simulink model "Quaternions_Method_main"  (R2021b)
settings: Solver=ode4  StartTime=0.0  StopTime=Time  FixedStep=1e-2  RelTol=1e-13  AbsTol=1e-8
values from neighbouring files (symbols this model uses):
  a = 8.6251e+06    (= 8625100)    [Main.m]
  c = 299792*10^3    (= 299792000)    [Main.m]
  e = 0.1195    [Main.m]
  f_mag = 5    [Main.m]
  H_0 = sqrt((g_1_0)^2 + (g_1_1)^2 + (h_1_1)^2)    [Main.m]
  i = 0.3815    [Main.m]
  MB = [2000; 0.3; 1; 0.12].*1e-2    [Main.m]
  mr = 1.2 * 0.0001    (= 0.00012)    [Main.m]
  muP = G*Mt    (= 398527110340000)    [Main.m]
  omega_0 = [om_x, om_y, om_z]    [Main.m]
  p_acc = deg2rad(5)    [Main.m]
  RD = 0.1*ones(1,10)    [Main.m]
  RS_MB = 0.5    [Main.m]
  RS_SP = 0.1    [Main.m]
  SP = [2000; 0.3; 1; 0.12].*1e-2    [Main.m]
  theta0 = 0    [Main.m]
  w_E = (2*pi)/(24*3600)    (= 7.27220521664e-05)    [Main.m]
undefined symbols (not defined in the file or in its folder): A_BN_0, A_rw, A_rw_star, k1, k2, magnitude, sig_b, sig_n, T, t_sample
libraries: matrix_library x15, vrlib x8, simulink x2, simulink_extras x1
(part 1 of 5)
settings Model: Creator=dario  LastModifiedBy=hp
settings SolverCC: ZeroCrossAlgorithm=Adaptive  AlgebraicLoopSolver=TrustRegion
settings DataIOCC: Refine=10
settings DebuggingCC: IgnoredZcDiagnostic=none

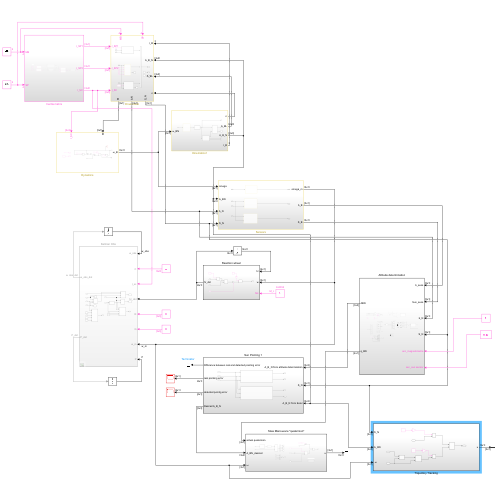
[thumbnail: Simulink's stored preview of the top-level diagram]
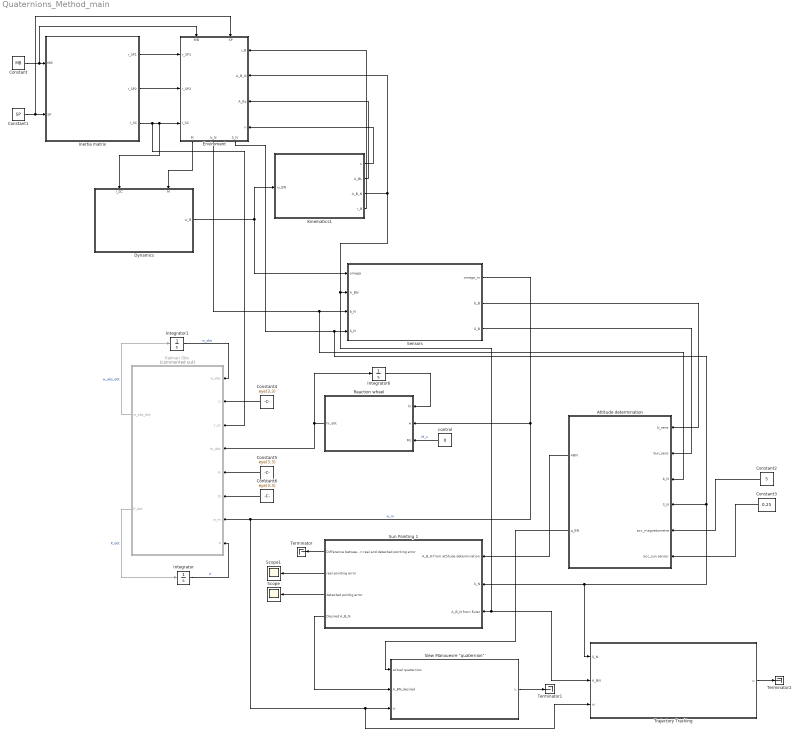
== system Quaternions_Method_main ==
  Attitude determination : Subsystem
  Constant : Constant  Value=MB
  Constant1 : Constant  Value=SP
  Constant2 : Constant  Value=5
  Constant3 : Constant  Value=0.25
  Constant4 : Constant  Value=eye(3,3)
  Constant5 : Constant  Value=eye(3,3)
  Constant6 : Constant  Value=eye(3,3)
  Dynamics : Subsystem
      settings: PortSchema="{\"entries\":[{\"content\":{\"sides\":[{\"content\":{\"connectorIds\":[]},\"type\":\"ConnectorPlacement.EquallySpacedRectSide\",\"uuid\":\"0fb0fd28-732a-45b7-951f-4b0b2306202c\"},{\"content\":{\"connectorIds\":[\"Out1\"],\"side\":\"RIGHT\"},\"type\":\"ConnectorPlacement.EquallySpacedRectSide\",\"uuid\":\"160a6d95-5e8b-4088-9ac4-372e2ef53b1e\"},{\"content\":{\"connectorIds\":[\"In1\",\"In2\"],\"side\":\"TOP\"},\"type\":\"ConnectorPlacement.EquallySpacedRectSide\",\"uuid\":\"bc0d773d-9b3c-40c2-804a-fc9efd6e220c\"}]},\"type\":\"ConnectorPlacement.EquallySpacedConnector\",\"uuid\":\"1f85a25c-c8d4-4d9d-9994-483d99135538\"}],\"packageUris\":[\"http://schema.mathworks.com/mf0/Connector/R2020b\"],\"version\":\"1.0\"}"
  Enviroment : Subsystem
      settings: PortSchema="{\"entries\":[{\"content\":{\"sides\":[{\"content\":{\"connectorIds\":[\"In1\",\"In2\"]},\"type\":\"ConnectorPlacement.EquallySpacedRectSide\",\"uuid\":\"77a65197-c5ef-4c05-af97-bd670bb59a1b\"},{\"content\":{\"connectorIds\":[\"Out1\",\"Out2\",\"Out3\"],\"side\":\"RIGHT\"},\"type\":\"ConnectorPlacement.EquallySpacedRectSide\",\"uuid\":\"f4905732-994b-44e8-915f-1f1165b6d340\"},{\"content\":{\"connectorIds\":[\"In3\",\"In4\",\"In5\"],\"side\":\"TOP\"},\"type\":\"ConnectorPlacement.EquallySpacedRectSide\",\"uuid\":\"dbb628bc-072b-4daa-a580-a056bf799753\"},{\"content\":{\"connectorIds\":[\"In6\",\"In7\",\"In8\",\"In9\"],\"side\":\"BOTTOM\"},\"type\":\"ConnectorPlacement.EquallySpacedRectSide\",\"uuid\":\"e6af6235-b92e-4098-9bbc-91b77f168ead\"}]},\"type\":\"ConnectorPlacement.EquallySpacedConnector\",\"uuid\":\"a4645f0d-8f51-4ba7-9ec5-d423e83ccc17\"}],\"packageUris\":[\"http://schema.mathworks.com/mf0/Connector/R2020b\"],\"version\":\"1.0\"}"
  Inertia matrix : Subsystem
  Integrator : Integrator
  Integrator1 : Integrator
  Integrator6 : Integrator  InitialCondition=[0;0;0;0]
  Kalman Obs : Subsystem  Commented=on
  Kinematics1 : Subsystem
  Reaction wheel : Subsystem
  Scope : Scope
  Scope1 : Scope
  Sensors : Subsystem
  "Slew Manouevre \"quaternion\"" : Subsystem
  Sun Pointing 1 : Subsystem
  Terminator : Terminator
  Terminator1 : Terminator
  Terminator2 : Terminator
  Trajectory Tracking : Subsystem
  control : Constant  Value=0
  wires:
  Constant6/1 -> Kalman Obs/6(Q)
  Sun Pointing 1/1(Difference between real and detected pointing error) -> Terminator/1
  Sun Pointing 1/2(real pointing error) -> Scope1/1
  Sensors/2(b_B) -> Attitude determination/1(b_sens)
  Integrator1/1 -> Kalman Obs/1(w_obs)  "w_obs"
  Enviroment/3(S_N) -> Trajectory Tracking/1(S_N), Sun Pointing 1/2(S_N), Attitude determination/4(S_N), Sensors/4(S_N)
  Inertia matrix/3(I_SC) -> Kalman Obs/3(I_sc), Enviroment/5(I_SC), Dynamics/1(I_SC)
  Integrator6/1 -> Reaction wheel/1(hr)
  Sun Pointing 1/3(detected pointig error) -> Scope/1
  Constant2/1 -> Attitude determination/5(acc_magnetometre)
  Sensors/3(S_B) -> Attitude determination/2(Sun_sens)
  Kalman Obs/1(w_obs_dot) -> Integrator1/1  "w_obs_dot"
  Dynamics/1(ω_B) -> Kinematics1/1(ω_BN), Sensors/1(omega)
  Enviroment/2(b_N) -> Attitude determination/3(b_N), Sensors/3(b_N)
  Constant4/1 -> Kalman Obs/2(C)
  Attitude determination/1(ABN) -> Sun Pointing 1/1(A_B_N from attitude determination)
  Inertia matrix/2(r_SP2) -> Enviroment/4(r_SP2)
  Constant3/1 -> Attitude determination/6(acc_sun sensor)
  Kinematics1/1(n) -> Enviroment/9(n)
  Constant5/1 -> Kalman Obs/5(R)
  control/1 -> Reaction wheel/3(Mc)  "M_c"
  Attitude determination/2(q_BN) -> "Slew Manouevre \"quaternion\""/1(actual quaternion)
  Inertia matrix/1(r_SP1) -> Enviroment/3(r_SP1)
  Constant1/1 -> Inertia matrix/2(SP), Enviroment/2(SP)
  Kinematics1/4(r_B) -> Enviroment/6(r_B)
  Reaction wheel/1(hr_dot) -> Integrator6/1, Kalman Obs/4(hr_dot)
  Sensors/1(omega_m) -> Reaction wheel/2(w), Trajectory Tracking/3(" ω"), "Slew Manouevre \"quaternion\""/3(ω), Kalman Obs/7(w_m)  "w_m"
  Constant/1 -> Inertia matrix/1(MB), Enviroment/1(MB)
  Kinematics1/3(A_B_N) -> Enviroment/7(A_B_N), Trajectory Tracking/2(A_BN), Sun Pointing 1/3(A_B_N from Euler), Sensors/2(A_BN)
  Enviroment/1(M) -> Dynamics/2(M)
  Kalman Obs/2(P_dot) -> Integrator/1  "P_dot"
  Integrator/1 -> Kalman Obs/8(P)  "P"
  Kinematics1/2(A_BL) -> Enviroment/8(A_BL)
  Sun Pointing 1/4(Desired A_B_N) -> "Slew Manouevre \"quaternion\""/2(A_BN_desired)
  "Slew Manouevre \"quaternion\""/1(u) -> Terminator1/1
  Trajectory Tracking/1(u) -> Terminator2/1

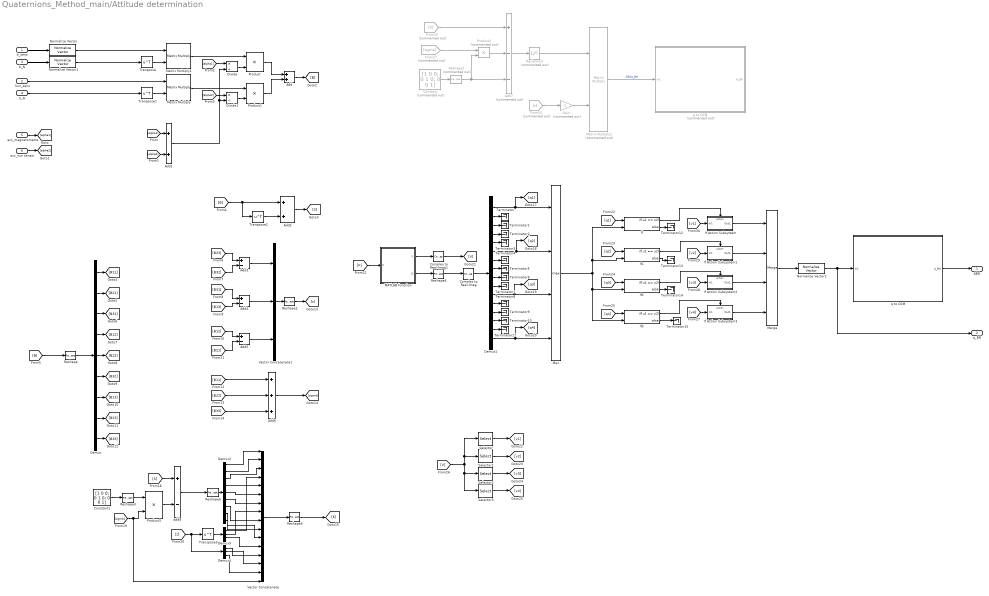
== system Quaternions_Method_main/Attitude determination ==
  b_sens : Inport
  Sun_sens : Inport  Port=2
  b_N : Inport  Port=3
  S_N : Inport  Port=4
  acc_magnetometre : Inport  Port=5
  acc_sun sensor : Inport  Port=6
  Add : Sum
  Add1 : Sum
  Add2 : Sum
  Add{3..5,8} (4 alike) : Sum  Inputs=+-
  Add6 : Sum  Inputs=+++
  Add7 : Sum  Commented=on  Inputs=+--
  Complex to Real-Imag : ComplexToRealImag  Output=Real
  Complex to Real-Imag1 : ComplexToRealImag  Output=Real
  Constant : Constant  Commented=on  Value=[1 0 0; 0 1 0; 0 0 1]  VectorParams1D=off
  Constant1 : Constant  Value=[1 0 0; 0 1 0; 0 0 1]  VectorParams1D=off
  Demux : Demux  Outputs=9
  Demux1 : Demux  Outputs=16
  Demux2 : Demux  Outputs=9
  Demux3 : Demux  Outputs=3
  Demux4 : Demux  Outputs=3
  Divide : Product  Inputs=*/
  Divide1 : Product  Inputs=*/
  From15 : From  Commented=on  GotoTag=z
  From16 : From  Commented=on  GotoTag=S
  From17 : From  Commented=on  GotoTag=sigma
  Gain : Gain  Commented=on  Gain=-1
  If{,1..3} (4 alike) : If  NumInputs=2  IfExpression=u1 == u2
  If Action Subsystem : Subsystem  TreatAsAtomicUnit=on
  If Action Subsystem1 : Subsystem  TreatAsAtomicUnit=on
  If Action Subsystem2 : Subsystem  TreatAsAtomicUnit=on
  If Action Subsystem3 : Subsystem  TreatAsAtomicUnit=on
  MATLAB Function : MATLAB Function  TreatAsAtomicUnit=on
  Matrix Multiply : Product  Multiplication=Matrix(*)
  Matrix Multiply1 : Product  Multiplication=Matrix(*)
  Matrix Multiply2 : Product  Commented=on  Multiplication=Matrix(*)
  Max : MinMax  Function=max  Inputs=4
  Merge : Merge  Inputs=4
  Normalize Vector : vrlib/Utilities/Normalize Vector  maxzero=0
  Normalize Vector1 : vrlib/Utilities/Normalize Vector  maxzero=0
  Normalize Vector2 : vrlib/Utilities/Normalize Vector  maxzero=0
  Product : Product
  Product1 : Product
  Product2 : Product  Commented=on
  Product3 : Product
  Reciprocal : Product  Commented=on  Inputs=/
  Reshape : Reshape
  Reshape1 : Reshape  OutputDimensionality=Column vector (2-D)
  Reshape2 : Reshape  Commented=on  OutputDimensionality=Customize  OutputDimensions=[3,3]
  Reshape3 : Reshape  OutputDimensionality=Customize  OutputDimensions=[3,3]
  Reshape4 : Reshape  OutputDimensionality=Column vector (2-D)
  Reshape5 : Reshape  OutputDimensionality=Column vector (2-D)
  Reshape6 : Reshape  OutputDimensionality=Customize  OutputDimensions=[4,4]
  Selector : Selector  NumberOfDimensions=2  InputPortWidth=3  IndexOptions=Index vector (dialog),Index vector (dialog)  Indices=[1 2 3 4],1  OutputSizes=1,1
  Selector1 : Selector  NumberOfDimensions=2  InputPortWidth=3  IndexOptions=Index vector (dialog),Index vector (dialog)  Indices=[1 2 3 4],2  OutputSizes=1,1
  Selector2 : Selector  NumberOfDimensions=2  InputPortWidth=3  IndexOptions=Index vector (dialog),Index vector (dialog)  Indices=[1 2 3 4],3  OutputSizes=1,1
  Selector3 : Selector  NumberOfDimensions=2  InputPortWidth=3  IndexOptions=Index vector (dialog),Index vector (dialog)  Indices=[1 2 3 4],4  OutputSizes=1,1
  Terminator{,1..15} (16 alike) : Terminator
  Transpose{,1..3} (4 alike) : Math  Operator=transpose  SaturateOnIntegerOverflow=on
  Vector Concatenate : Concatenate  NumInputs=16
  Vector Concatenate1 : Concatenate  NumInputs=3
  g to DCM : Subsystem  Commented=on
  q to DCM : Subsystem
  ABN : Outport
  q_BN : Outport  Port=2
  wires:
  b_N/1 -> Normalize Vector1/1
  S_N/1 -> Transpose1/1
  Sun_sens/1 -> Matrix Multiply/1
  Transpose1/1 -> Matrix Multiply/2
  Transpose/1 -> Matrix Multiply1/2
  b_sens/1 -> Normalize Vector/1
  Matrix Multiply1/1 -> Product/1
  Product/1 -> Add/1
  Divide/1 -> Product/2
  Divide1/1 -> Product1/2
  Product1/1 -> Add/2
  Matrix Multiply/1 -> Product1/1
  Add1/1 -> Divide/2, Divide1/2
  acc_magnetometre/1 -> [alpha1]
  acc_sun sensor/1 -> [alpha2]
  [alpha1] -> Add1/1
  [alpha2] -> Add1/2
  [alpha2] -> Divide1/1
  [alpha1] -> Divide/1
  Add/1 -> [B]
  [B] -> Transpose2/1, Add2/1
  Transpose2/1 -> Add2/2
  Add2/1 -> [S]
  [B] -> Reshape/1
  Reshape/1 -> Demux/1
  Demux/1 -> [B11]
  Demux/2 -> [B21]
  Demux/3 -> [B31]
  Demux/4 -> [B12]
  Demux/5 -> [B22]
  Demux/6 -> [B32]
  Demux/7 -> [B13]
  Demux/8 -> [B23]
  Demux/9 -> [B33]
  [B23] -> Add3/1
  [B32] -> Add3/2
  [B31] -> Add4/1
  [B13] -> Add4/2
  [B12] -> Add5/1
  [B21] -> Add5/2
  Add3/1 -> Vector Concatenate1/1
  Add4/1 -> Vector Concatenate1/2
  Add5/1 -> Vector Concatenate1/3
  Vector Concatenate1/1 -> Reshape1/1
  Reshape1/1 -> [z]
  [B11] -> Add6/1
  [B22] -> Add6/2
  [B33] -> Add6/3
  Add6/1 -> [sigma]
  From15/1 -> Gain/1
  Constant/1 -> Reshape2/1
  From17/1 -> Product2/1
  Reshape2/1 -> Add7/3, Product2/2
  From16/1 -> Add7/1
  Product2/1 -> Add7/2
  Add7/1 -> Reciprocal/1
  Reciprocal/1 -> Matrix Multiply2/1
  Gain/1 -> Matrix Multiply2/2
  Matrix Multiply2/1 -> g to DCM/1(In1)  "Gibbs_BN"
  Constant1/1 -> Reshape3/1
  Reshape3/1 -> Product3/1
  [sigma] -> Vector Concatenate/16, Product3/2
  Product3/1 -> Add8/2
  [S] -> Add8/1
  Add8/1 -> Reshape5/1
  MATLAB Function/2(D) -> Reshape4/1
  Demux1/2 -> Terminator/1
  Demux1/3 -> Terminator1/1
  Demux1/4 -> Terminator2/1
  Demux1/5 -> Terminator3/1
  Demux1/6 -> [q2], Max/2
  Demux1/7 -> Terminator4/1
  Demux1/8 -> Terminator5/1
  Demux1/9 -> Terminator6/1
  Demux1/10 -> Terminator7/1
  Demux1/11 -> [q3], Max/3
  Demux1/16 -> [q4], Max/4
  Demux1/12 -> Terminator8/1
  Demux1/13 -> Terminator9/1
  Demux1/14 -> Terminator10/1
  Demux1/15 -> Terminator11/1
  Reshape4/1 -> Complex to Real-Imag/1
  Max/1 -> If3/2, If2/2, If1/2, If/2
  Demux1/1 -> [q1], Max/1
  [q1] -> If/1
  [q2] -> If1/1
  [q4] -> If3/1
  [q3] -> If2/1
  MATLAB Function/1(V) -> Complex to Real-Imag1/1
  Selector1/1 -> [v2]
  Selector3/1 -> [v4]
  Selector2/1 -> [v3]
  Selector/1 -> [v1]
  [V] -> Selector/1, Selector1/1, Selector3/1, Selector2/1
  If/1 -> If Action Subsystem/Action
  If/2 -> Terminator12/1
  If1/2 -> Terminator13/1
  If2/2 -> Terminator14/1
  If3/2 -> Terminator15/1
  If Action Subsystem/1(Out1) -> Merge/1
  If1/1 -> If Action Subsystem1/Action
  If2/1 -> If Action Subsystem2/Action
  If3/1 -> If Action Subsystem3/Action
  If Action Subsystem3/1(Out1) -> Merge/4
  If Action Subsystem2/1(Out1) -> Merge/3
  If Action Subsystem1/1(Out1) -> Merge/2
  [v4] -> If Action Subsystem3/1(In1)
  [v1] -> If Action Subsystem/1(In1)
  [v2] -> If Action Subsystem1/1(In1)
  Normalize Vector/1 -> Matrix Multiply1/1
  Normalize Vector1/1 -> Transpose/1
  [v3] -> If Action Subsystem2/1(In1)
  q to DCM/1(A_BN) -> ABN/1
  Merge/1 -> Normalize Vector2/1
  Reshape5/1 -> Demux2/1
  Demux2/1 -> Vector Concatenate/1
  Demux2/2 -> Vector Concatenate/2
  Demux2/3 -> Vector Concatenate/3
  [z] -> Demux4/1, Transpose3/1
  Transpose3/1 -> Demux3/1
  Demux3/1 -> Vector Concatenate/4
  Demux2/4 -> Vector Concatenate/5
  Demux2/5 -> Vector Concatenate/6
  Demux2/6 -> Vector Concatenate/7
  Demux3/2 -> Vector Concatenate/8
  Demux2/7 -> Vector Concatenate/9
  Demux2/8 -> Vector Concatenate/10
  Demux2/9 -> Vector Concatenate/11
  Demux3/3 -> Vector Concatenate/12
  Demux4/2 -> Vector Concatenate/14
  Demux4/1 -> Vector Concatenate/13
  Demux4/3 -> Vector Concatenate/15
  Vector Concatenate/1 -> Reshape6/1
  Reshape6/1 -> [K]
  Complex to Real-Imag/1 -> Demux1/1
  Normalize Vector2/1 -> q_BN/1, q to DCM/1(In1)
  Complex to Real-Imag1/1 -> [V]
  [K] -> MATLAB Function/1(K)

== system Quaternions_Method_main/Dynamics ==
  I_SC : Inport
  M : Inport  Port=2
  Constant7 : Constant  Value=omega_0
  Cross Product : vrlib/Utilities/Cross Product
  Gain5 : Gain  Gain=-1
  Integrator4 : Integrator  InitialConditionSource=external  InitialCondition=omega_0
  Product6 : Product  Multiplication=Matrix(*)
  Product7 : Product  Multiplication=Matrix(*)
  Reciprocal : Product  Inputs=/  Multiplication=Matrix(*)
  Scope : Scope
  Sum2 : Sum
  Terminator : Terminator
  ω_B : Outport
  wires:
  Sum2/1 -> Product7/2
  Product6/1 -> Cross Product/2
  Product7/1 -> Terminator/1, Integrator4/1
  Cross Product/1 -> Gain5/1
  Gain5/1 -> Sum2/1
  Integrator4/1 -> Scope/1, Cross Product/1, Product6/2, ω_B/1
  I_SC/1 -> [I_SC]
  [I_SC] -> Product6/1
  [I_SC] -> Reciprocal/1
  Reciprocal/1 -> Product7/1
  Constant7/1 -> [w_0]
  [w_0] -> Integrator4/2
  M/1 -> Sum2/2

== system Quaternions_Method_main/Enviroment ==
  MB : Inport
  SP : Inport  Port=2
  r_SP1 : Inport  Port=3
  r_SP2 : Inport  Port=4
  I_SC : Inport  Port=5
  r_B : Inport  Port=6
  A_B_N : Inport  Port=7
  A_BL : Inport  Port=8
  n : Inport  Port=9
  Constant : Constant  Value=6371.2*1e3
  Gravity gradient torque : Subsystem
  "Magnetic torque " : Subsystem
  Solar Radiation Perturbation : Subsystem
  Sum : Sum  Inputs=+|+|+
  M : Outport
  b_N : Outport  Port=2
  S_N : Outport  Port=3
  wires:
  A_B_N/1 -> "Magnetic torque "/3(A_B_N), Solar Radiation Perturbation/1(A_B_N)
  MB/1 -> Solar Radiation Perturbation/2(MB)
  SP/1 -> Solar Radiation Perturbation/3(SP)
  r_SP1/1 -> Solar Radiation Perturbation/4(r_SP1)
  r_SP2/1 -> Solar Radiation Perturbation/5(r_SP2)
  Sum/1 -> M/1
  Solar Radiation Perturbation/1(M_SRP) -> Sum/2
  "Magnetic torque "/1(M) -> Sum/3
  r_B/1 -> "Magnetic torque "/1(r_B)
  Constant/1 -> "Magnetic torque "/2(R)
  Gravity gradient torque/1(M_GG) -> Sum/1
  I_SC/1 -> Gravity gradient torque/1(I)
  n/1 -> Gravity gradient torque/3(n)
  A_BL/1 -> Gravity gradient torque/2(A_BL)
  "Magnetic torque "/2(b_N) -> [b_N]
  [b_N] -> b_N/1
  Solar Radiation Perturbation/2(S_N) -> [S_N]
  [S_N] -> S_N/1

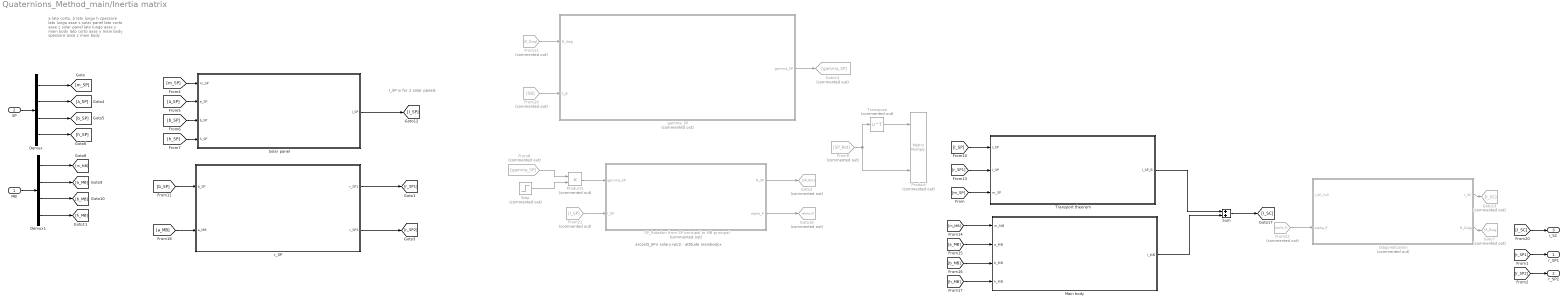
== system Quaternions_Method_main/Inertia matrix ==
  note: I_SP is for 2 solar panels
  note: arcos(S_B*n solary)-pi/2 - attitude mainbodyx
  note: a lato corto, b lato lungo h spessore
      | lato lungo asse x solar panel
      | lato corto asse z solar panel
      | lato lungo asse y main body
      | lato corto asse x main body
      | spessore asse z main body
  MB : Inport
  SP : Inport  Port=2
  Demux : Demux
  Demux1 : Demux
  Diagonalization : Subsystem  Commented=on
  From12 : From  Commented=on  GotoTag=R_Diag
  From19 : From  Commented=on  GotoTag=SB
  From21 : From  Commented=on  GotoTag=I_SP
  From22 : From  Commented=on  GotoTag=alpha_P
  From8 : From  Commented=on  GotoTag=gamma_SP
  From9 : From  Commented=on  GotoTag=SP_Rot
  Goto13 : Goto  Commented=on  GotoTag=I_SC
  Goto14 : Goto  Commented=on  GotoTag=gamma_SP
  Goto16 : Goto  Commented=on  GotoTag=alpha_P
  Goto2 : Goto  Commented=on  GotoTag=SP_Rot
  Goto7 : Goto  Commented=on  GotoTag=R_Diag
  Main body : Subsystem
  Product : Product  Commented=on  Inputs=3  Multiplication=Matrix(*)
  Product1 : Product  Commented=on
  SP_Rotation from SP principal to MB principal : Subsystem  Commented=on
  Solar panel : Subsystem
  Step : Step  Commented=on  Time=1e-3  SampleTime=0
  Sum : Sum
  Transport theorem : Subsystem
  Transpose : Math  Commented=on  Operator=transpose  SaturateOnIntegerOverflow=on
  gamma_SP : Subsystem  Commented=on
  r_SP : Subsystem
  r_SP1 : Outport
  r_SP2 : Outport  Port=2
  I_SC : Outport  Port=3
  wires:
  MB/1 -> Demux1/1
  Demux/1 -> [m_SP]
  SP_Rotation from SP principal to MB principal/1(R_SP) -> Goto2/1
  Transpose/1 -> Product/1
  Transport theorem/1(I_SP_B) -> Sum/1
  [r_SP1] -> Transport theorem/2(r_SP)
  Main body/1(I_MB) -> Sum/2
  [m_SP] -> Transport theorem/3(m_SP)
  r_SP/1(r_SP1) -> [r_SP1]
  [r_SP1] -> r_SP1/1
  [r_SP2] -> r_SP2/1
  r_SP/2(r_SP2) -> [r_SP2]
  Demux/2 -> [a_SP]
  Demux/3 -> [b_SP]
  Demux/4 -> [h_SP]
  [a_SP] -> Solar panel/2(a_SP)
  [b_SP] -> Solar panel/3(b_SP)
  [m_SP] -> Solar panel/1(m_SP)
  [h_SP] -> Solar panel/4(h_SP)
  From9/1 -> Transpose/1, Product/3
  [b_SP] -> r_SP/1(b_SP)
  Demux1/4 -> [h_MB]
  Demux1/3 -> [b_MB]
  Demux1/2 -> [a_MB]
  Demux1/1 -> [m_MB]
  [m_MB] -> Main body/1(m_MB)
  [a_MB] -> Main body/2(a_MB)
  [b_MB] -> Main body/3(b_MB)
  [h_MB] -> Main body/4(h_MB)
  [a_MB] -> r_SP/2(a_MB)
  Solar panel/1(I_SP) -> [I_SP]
  Product1/1 -> SP_Rotation from SP principal to MB principal/1(gamma_SP)
  From8/1 -> Product1/1
  Step/1 -> Product1/2
  SP/1 -> Demux/1
  Diagonalization/2(R_Diag) -> Goto7/1
  From12/1 -> gamma_SP/1(R_diag)
  From19/1 -> gamma_SP/2(S_B)
  Diagonalization/1(I_SC) -> Goto13/1
  [I_SC] -> I_SC/1
  gamma_SP/1(gamma_SP) -> Goto14/1
  From21/1 -> SP_Rotation from SP principal to MB principal/2(I_SP)
  SP_Rotation from SP principal to MB principal/2(alpha_P) -> Goto16/1
  From22/1 -> Diagonalization/2(alpha_P)
  [I_SP] -> Transport theorem/1(I_SP)
  Sum/1 -> [I_SC]

== system Quaternions_Method_main/Kalman Obs ==
  w_obs : Inport
  C : Inport  Port=2
  I_sc : Inport  Port=3
  hr_dot : Inport  Port=4
  R : Inport  Port=5
  Q : Inport  Port=6
  w_m : Inport  Port=7
  P : Inport  Port=8
  Subsystem : Subsystem
  Subsystem1 : Subsystem
  Subsystem2 : Subsystem
  Subsystem3 : Subsystem
  Subsystem4 : Subsystem
  Subsystem5 : Subsystem
  w_obs_dot : Outport
  P_dot : Outport  Port=2
  wires:
  I_sc/1 -> Subsystem4/3(I_sc), Subsystem/1(I_SC)
  Subsystem/1(K) -> Subsystem4/1(K), Subsystem1/2(K)  "K"
  w_obs/1 -> Subsystem4/2(w_obs), Subsystem1/1(w_obs), Subsystem3/4(w_obs)
  Subsystem1/1(A) -> [A]
  C/1 -> Subsystem3/3(C), [C], Subsystem2/1(C)
  P/1 -> Subsystem5/1(P), Subsystem2/2(P)
  R/1 -> Subsystem2/3(R), [R]
  Subsystem2/1(L) -> Subsystem3/1(L)  "L"
  w_m/1 -> Subsystem3/2(w_m)
  Subsystem3/1(Ly) -> [Ly]
  Subsystem4/1(w_obs_dot) -> w_obs_dot/1
  hr_dot/1 -> Subsystem4/4(hr_dot)
  [Ly] -> Subsystem4/5(Ly)
  [A] -> Subsystem5/2(A)
  Q/1 -> Subsystem5/3(Q)
  [C] -> Subsystem5/4(C)
  [R] -> Subsystem5/5(R)
  Subsystem5/1(P_dot) -> P_dot/1

== system Quaternions_Method_main/Kinematics1 ==
  ω_BN : Inport
  Creazione Matrice A_BN : Subsystem
  Creazione quaternione : Subsystem
  Orbit Propagation : Subsystem
  Relative_Attitude : Subsystem
  n : Outport
  A_BL : Outport  Port=2
  A_B_N : Outport  Port=3
  r_B : Outport  Port=4
  wires:
  Creazione Matrice A_BN/1(A_BN) -> A_B_N/1, Relative_Attitude/1(A_BN), Orbit Propagation/1(A_BN)
  ω_BN/1 -> Creazione quaternione/1(ω_BN)
  Creazione quaternione/1(q_normalizzato) -> Creazione Matrice A_BN/1(q_normalizzato)
  Relative_Attitude/1(A_BL) -> A_BL/1
  Orbit Propagation/2(n) -> n/1
  Orbit Propagation/3(rB) -> r_B/1
  Orbit Propagation/1(theta) -> Relative_Attitude/2(theta)
  Relative_Attitude/2(A_L/N) -> [A_LN]

== system Quaternions_Method_main/Reaction wheel ==
  hr : Inport
  w : Inport  Port=2
  Mc : Inport  Port=3
  A : Constant  Value=A_rw
  A_star : Constant  Value=A_rw_star
  Cross Product : matrix_library/Cross Product
      settings: SourceProductBaseCode=SL
  Gain : Gain  Gain=-1
  Matrix Multiply : Product  Multiplication=Matrix(*)
  Matrix Multiply1 : Product  Multiplication=Matrix(*)
  Sum : Sum  Inputs=|++
  hr_dot : Outport
  wires:
  hr/1 -> Matrix Multiply/2
  A/1 -> Matrix Multiply/1
  w/1 -> Cross Product/1
  Matrix Multiply/1 -> Cross Product/2
  Cross Product/1 -> Sum/1
  Mc/1 -> Sum/2
  Sum/1 -> Matrix Multiply1/2
  A_star/1 -> Gain/1
  Gain/1 -> Matrix Multiply1/1
  Matrix Multiply1/1 -> hr_dot/1

== system Quaternions_Method_main/Sensors ==
  omega : Inport
  A_BN : Inport  Port=2
  b_N : Inport  Port=3
  S_N : Inport  Port=4
  Gyroscopes : Subsystem
  Magnetometer1 : Subsystem
  Sun sensor : Subsystem
  omega_m : Outport
  b_B : Outport  Port=2
  S_B : Outport  Port=3
  wires:
  omega/1 -> Gyroscopes/1(omega)
  Gyroscopes/1(omega_m) -> omega_m/1
  b_N/1 -> Magnetometer1/2(b_N)
  Magnetometer1/1(b_B) -> b_B/1
  Sun sensor/1(S_B) -> S_B/1
  A_BN/1 -> Sun sensor/2(A_BN), Magnetometer1/1(A_BN)
  S_N/1 -> Sun sensor/1(S_N)

== system Quaternions_Method_main/Slew Manouevre "quaternion" ==
  note: here I compute the derivative wrt q4e
      | of the function H(q4e) = 1 - q4e^2
  actual quaternion : Inport
  A_BN_desired : Inport  Port=2
  ω : Inport  Port=3
  A_BN to quaternion : Subsystem
  Constant : Constant  Value=k1
  Constant1 : Constant  Value=k2
  Creation of Q_euler1 : Subsystem
  Demux : Demux
  Gain : Gain  Gain=-1
  Gain1 : Gain  Gain=-2
  Mux : Mux  Inputs=3
  Product : Product  Multiplication=Matrix(*)
  Product1 : Product
  Product2 : Product  Inputs=3
  Reshape : Reshape  OutputDimensionality=Column vector (2-D)
  Sum : Sum  Inputs=|+|+|
  d/dq4e(H(q4e)) : Subsystem  Commented=on
  u : Outport
  wires:
  actual quaternion/1 -> Product/2
  Creation of Q_euler1/1(Q_desired) -> Product/1
  A_BN_desired/1 -> A_BN to quaternion/1(" A_BN_Desiderd")
  A_BN to quaternion/1(q_desiderd) -> Creation of Q_euler1/1(q_desired)
  Constant/1 -> Gain/1
  Gain/1 -> Product1/1
  ω/1 -> Product1/2
  Constant1/1 -> Product2/1
  [q_error] -> Product2/3
  Product1/1 -> Sum/1
  Product2/1 -> Sum/2
  Sum/1 -> u/1
  Product/1 -> Demux/1
  Demux/1 -> [qe1]
  Demux/4 -> [qe4]
  Demux/3 -> [qe3]
  Demux/2 -> [qe2]
  [qe1] -> Mux/1
  [qe2] -> Mux/2
  [qe3] -> Mux/3
  Mux/1 -> Reshape/1
  Reshape/1 -> [q_error]
  [qe4] -> Gain1/1
  Gain1/1 -> Product2/2

== system Quaternions_Method_main/Sun Pointing 1 ==
  A_B_N from attitude determination : Inport
  S_N : Inport  Port=2
  A_B_N from Euler : Inport  Port=3
  Pointing error with DCM : Subsystem
  Pointing error with quaternions : Subsystem
  Difference between real and detected pointing error : Outport
  real pointing error : Outport  Port=2
  detected pointig error : Outport  Port=3
  Desired A_B_N : Outport  Port=4
  wires:
  A_B_N from attitude determination/1 -> Pointing error with quaternions/1(A_B_N from attitude determination), Pointing error with DCM/3(A_B_N from Euler)
  S_N/1 -> Pointing error with quaternions/2(S_N), Pointing error with DCM/2(S_N)
  A_B_N from Euler/1 -> Pointing error with quaternions/3(A_B_N from Euler), Pointing error with DCM/1(A_B_N from attitude determination)
  Pointing error with DCM/1(Difference between real and detected pointing error) -> Difference between real and detected pointing error/1
  Pointing error with quaternions/2(detected pointing error) -> detected pointig error/1
  Pointing error with quaternions/1(real pointing error) -> real pointing error/1
  Pointing error with DCM/2(Desired A_B_N) -> Desired A_B_N/1

== system Quaternions_Method_main/Trajectory Tracking ==
  S_N : Inport
  A_BN : Inport  Port=2
  " ω" : Inport  Port=3
  Constant : Constant  Value=k1
  Constant1 : Constant  Value=k2
  Cross Product : matrix_library/Cross Product
      settings: SourceProductBaseCode=SL
  Gain : Gain  Gain=-1
  Gain1 : Gain  Gain=-1
  Matrix Multiply : Product  Multiplication=Matrix(*)
  Product : Product
  Product1 : Product
  Sum : Sum  Inputs=|+|+|
  u : Outport
  wires:
  S_N/1 -> Cross Product/2, Matrix Multiply/2
  A_BN/1 -> Matrix Multiply/1
  Constant/1 -> Gain/1
  Constant1/1 -> Gain1/1
  Matrix Multiply/1 -> Cross Product/1
  Cross Product/1 -> Product/2
  Gain1/1 -> Product/1
  Gain/1 -> Product1/1
  " ω"/1 -> Product1/2
  Product1/1 -> Sum/1
  Product/1 -> Sum/2
  Sum/1 -> u/1

== system Quaternions_Method_main/Attitude determination/If Action Subsystem ==
  In1 : Inport
  Action Port : ActionPort  ActionPortLabel=if(u1 == u2)
  Out1 : Outport
  wires:
  In1/1 -> Out1/1

== system Quaternions_Method_main/Attitude determination/If Action Subsystem1 ==
  In1 : Inport
  Action Port : ActionPort  ActionPortLabel=if(u1 == u2)
  Out1 : Outport
  wires:
  In1/1 -> Out1/1

== system Quaternions_Method_main/Attitude determination/If Action Subsystem2 ==
  In1 : Inport
  Action Port : ActionPort  ActionPortLabel=if(u1 == u2)
  Out1 : Outport
  wires:
  In1/1 -> Out1/1

== system Quaternions_Method_main/Attitude determination/If Action Subsystem3 ==
  In1 : Inport
  Action Port : ActionPort  ActionPortLabel=if(u1 == u2)
  Out1 : Outport
  wires:
  In1/1 -> Out1/1

== system Quaternions_Method_main/Attitude determination/g to DCM ==
  In1 : Inport
  A_BN : Outport
  wires:
  In1/1 -> A_BN/1

== system Quaternions_Method_main/Attitude determination/q to DCM ==
  In1 : Inport
  Add : Sum  Inputs=+-
  Add1 : Sum  Inputs=++-
  Constant : Constant  Value=[1 0 0; 0 1 0; 0 0 1]  VectorParams1D=off
  Demux : Demux
  Gain : Gain  Gain=2
  Gain1 : Gain  Gain=2
  Matrix Multiply : Product  Multiplication=Matrix(*)
  Matrix Multiply2 : Product  Multiplication=Matrix(*)
  Mux : Mux  Inputs=3
  Product : Product
  Product1 : Product
  Reshape : Reshape  OutputDimensionality=Column vector (2-D)
  Reshape1 : Reshape  OutputDimensionality=Customize  OutputDimensions=[3,3]
  Square : Math  Operator=square  SaturateOnIntegerOverflow=on
  Transpose : Math  Operator=transpose  SaturateOnIntegerOverflow=on
  Transpose1 : Math  Operator=transpose  SaturateOnIntegerOverflow=on
  q_cross : Subsystem
  A_BN : Outport
  wires:
  In1/1 -> Demux/1
  Demux/4 -> [q4]
  Demux/1 -> [q1]
  Demux/2 -> [q2]
  Demux/3 -> [q3]
  [q4] -> Square/1
  [q2] -> Mux/2
  [q3] -> Mux/3
  [q1] -> Mux/1
  Mux/1 -> Reshape/1
  Reshape/1 -> [q_vect]
  [q_vect] -> Matrix Multiply/2, Transpose/1
  Transpose/1 -> Matrix Multiply/1
  Matrix Multiply/1 -> Add/2
  Square/1 -> Add/1
  Constant/1 -> Reshape1/1
  Reshape1/1 -> Product1/2
  Product1/1 -> Add1/1
  Matrix Multiply2/1 -> Gain/1
  Gain/1 -> Add1/2
  Transpose1/1 -> Matrix Multiply2/2
  [q_vect] -> Transpose1/1, Matrix Multiply2/1
  Gain1/1 -> Add1/3
  Product/1 -> Gain1/1
  [q4] -> Product/2
  q_cross/1(q_cross) -> Product/1
  Add1/1 -> A_BN/1
  [q_vect] -> q_cross/1(q_vect)
  Add/1 -> Product1/1

== system Quaternions_Method_main/Enviroment/Gravity gradient torque ==
  I : Inport
  A_BL : Inport  Port=2
  n : Inport  Port=3
  Constant1 : Constant  Value=[1 0 0]
  Demux : Demux  Outputs=9
  Demux1 : Demux  Outputs=3
  Matrix Multiply : Product  Multiplication=Matrix(*)
  Mux : Mux  Inputs=3
  Product{1..9} (9 alike) : Product
  Reshape : Reshape  OutputDimensionality=Column vector (2-D)
  Reshape1 : Reshape  OutputDimensionality=Column vector (2-D)
  Sum : Sum  Inputs=+-
  Sum1 : Sum  Inputs=+-
  Sum2 : Sum  Inputs=+-
  Terminator{,1..5} (6 alike) : Terminator
  M_GG : Outport
  wires:
  Demux/4 -> Terminator2/1
  n/1 -> Product3/2, Product1/2, Product2/2
  Demux1/1 -> Product5/2, Product7/2
  Demux/2 -> Terminator/1
  Product6/1 -> Product9/1
  Sum/1 -> Product1/1
  Product1/1 -> Product6/1
  Demux/7 -> Terminator4/1
  Demux1/3 -> Product6/2, Product8/2
  Demux/1 -> Sum1/1
  Product5/1 -> Product8/1
  Demux/3 -> Terminator1/1
  I/1 -> Reshape1/1
  Matrix Multiply/1 -> Demux1/1
  Demux/9 -> Sum2/2, Sum1/2, Sum/1
  Constant1/1 -> Reshape/1
  Sum1/1 -> Product2/1
  Sum2/1 -> Product3/1
  Product7/1 -> Mux/3
  Mux/1 -> M_GG/1
  Demux/5 -> Sum/2, Sum2/1
  Demux/8 -> Terminator5/1
  A_BL/1 -> Matrix Multiply/1
  Product4/1 -> Product7/1
  Product8/1 -> Mux/2
  Demux/6 -> Terminator3/1
  Demux1/2 -> Product4/2, Product9/2
  Product2/1 -> Product5/1
  Product9/1 -> Mux/1
  Product3/1 -> Product4/1
  Reshape/1 -> Matrix Multiply/2
  Reshape1/1 -> Demux/1

== system Quaternions_Method_main/Enviroment/Magnetic torque  ==
  r_B : Inport
  R : Inport  Port=2
  A_B_N : Inport  Port=3
  Creation of parasitic torque : Subsystem
  Cross Product : matrix_library/Cross Product
      settings: SourceProductBaseCode=SL
  Magnetic torque in body frame : Subsystem
  Matrix Multiply : Product  Multiplication=Matrix(*)
  M : Outport
  b_N : Outport  Port=2
  wires:
  R/1 -> Magnetic torque in body frame/3(R)
  A_B_N/1 -> Magnetic torque in body frame/1(A_B_N), Matrix Multiply/1
  Magnetic torque in body frame/1(b_B) -> Cross Product/2
  Cross Product/1 -> M/1
  Matrix Multiply/1 -> Magnetic torque in body frame/2(r_N)
  r_B/1 -> Matrix Multiply/2
  Creation of parasitic torque/1(m) -> Cross Product/1
  Magnetic torque in body frame/2(b_N) -> b_N/1

== system Quaternions_Method_main/Enviroment/Solar Radiation Perturbation ==
  A_B_N : Inport
  MB : Inport  Port=2
  SP : Inport  Port=3
  r_SP1 : Inport  Port=4
  r_SP2 : Inport  Port=5
  Force1 : Subsystem
  Normalize Vector : vrlib/Utilities/Normalize Vector  maxzero=0
  Sum forces : Subsystem
      settings: PortSchema="{\"entries\":[{\"content\":{\"sides\":[{\"content\":{\"connectorIds\":[\"In1\",\"In2\",\"In3\",\"In4\",\"In5\",\"In6\",\"In7\"]},\"type\":\"ConnectorPlacement.EquallySpacedRectSide\",\"uuid\":\"5acb7d4f-0337-4224-9758-4598a3a00165\"},{\"content\":{\"connectorIds\":[\"Out1\"],\"side\":\"RIGHT\"},\"type\":\"ConnectorPlacement.EquallySpacedRectSide\",\"uuid\":\"e6f98c05-9b5f-4378-b9e9-dabff353d596\"},{\"content\":{\"connectorIds\":[],\"side\":\"TOP\"},\"type\":\"ConnectorPlacement.EquallySpacedRectSide\",\"uuid\":\"88e90ea7-7ab4-48d4-8e3b-8712b3a0b993\"},{\"content\":{\"connectorIds\":[\"In8\"],\"side\":\"BOTTOM\"},\"type\":\"ConnectorPlacement.EquallySpacedRectSide\",\"uuid\":\"ececea6a-2c27-462e-a638-503b4beb3cbf\"}]},\"type\":\"ConnectorPlacement.EquallySpacedConnector\",\"uuid\":\"86da1db6-5ce7-4d9e-9b5c-c43957a7360d\"}],\"packageUris\":[\"http://schema.mathworks.com/mf0/Connector/R2020b\"],\"version\":\"1.0\"}"
  Sun position body : Subsystem
  M_SRP : Outport
  S_N : Outport  Port=2
  wires:
  A_B_N/1 -> Sun position body/1(A_B_N)
  Sun position body/1(S_B) -> Normalize Vector/1
  Normalize Vector/1 -> Force1/1(SB)
  Force1/3(A_MB) -> Sum forces/5(A_MB)
  Force1/1(F_MB) -> Sum forces/3(F_MB)
  r_SP1/1 -> Sum forces/1(r_SP1)
  r_SP2/1 -> Sum forces/2(r_SP2)
  Force1/5(prodscal_SP1) -> Sum forces/7(prodscal_SP (tra norm e sun direction))
  Force1/4(prodsca_MB) -> Sum forces/6(prodscal_MB(tra norm e sun direction))
  Sum forces/1(M_SRP) -> M_SRP/1
  MB/1 -> [MB]
  SP/1 -> [SP]
  [MB] -> Force1/2(MB)
  [SP] -> Force1/3(SP)
  [MB] -> Sum forces/8(MB)
  Force1/2(F_SP) -> Sum forces/4(F_SP)
  Sun position body/2(S_N) -> [S_N]
  [S_N] -> S_N/1

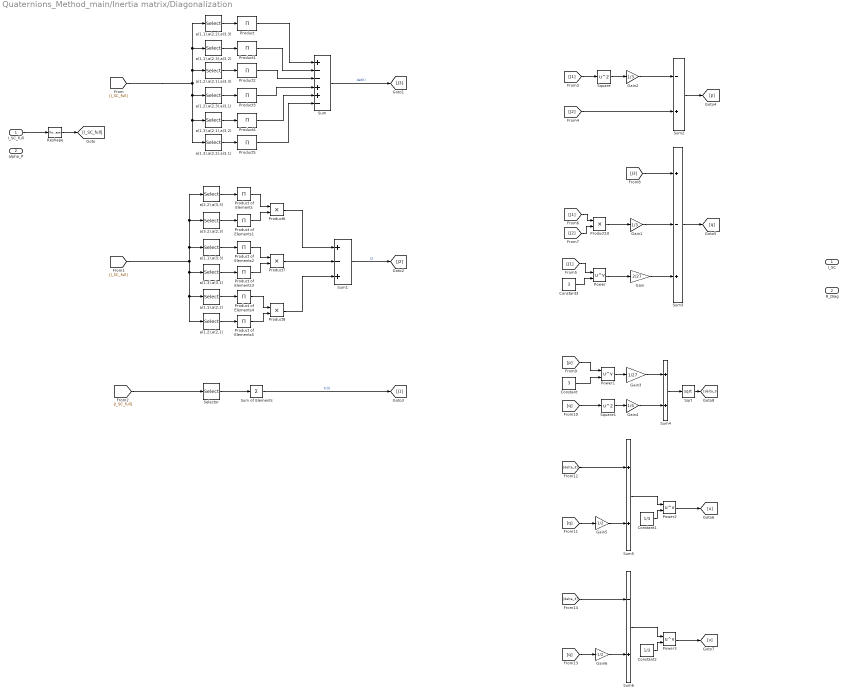
== system Quaternions_Method_main/Inertia matrix/Diagonalization ==
  I_SC_full : Inport
  alpha_P : Inport  Port=2
  Constant : Constant  Value=3
  Constant1 : Constant  Value=1/3
  Constant2 : Constant  Value=1/3
  Constant3 : Constant  Value=3
  Gain : Gain  Gain=2/27
  Gain1 : Gain  Gain=1/3
  Gain2 : Gain  Gain=1/3
  Gain3 : Gain  Gain=1/27
  Gain4 : Gain  Gain=1/4
  Gain5 : Gain  Gain=-1/2
  Gain6 : Gain  Gain=-1/2
  Power{,1..3} (4 alike) : Math  Operator=pow  SaturateOnIntegerOverflow=on
  Product{,1..5} (6 alike) : Product  Inputs=1  SaturateOnIntegerOverflow=on  OutDataTypeStr=Inherit: Same as first input
  Product of Elements{,1..5} (6 alike) : Product  Inputs=*
  Product{6..8,10} (4 alike) : Product
  Reshape : Reshape  OutputDimensionality=Column vector (2-D)
  Selector : Selector  InputPortWidth=9  IndexOptions=Index vector (dialog)  Indices=[1 5 9]  OutputSizes=1
  Sqrt : Sqrt  SaturateOnIntegerOverflow=on
  Square : Math  Operator=square  SaturateOnIntegerOverflow=on
  Square1 : Math  Operator=square  SaturateOnIntegerOverflow=on
  Sum : Sum  Inputs=+--++-  SaturateOnIntegerOverflow=on
  Sum of Elements : Sum  Inputs=+
  Sum1 : Sum  Inputs=+-+
  Sum2 : Sum  Inputs=-+
  Sum3 : Sum  Inputs=+-+
  Sum4 : Sum
  Sum5 : Sum
  Sum6 : Sum  Inputs=-+
  a(1,1),a(2,2) : Selector  InputPortWidth=9  IndexOptions=Index vector (dialog)  Indices=[1 3]  OutputSizes=1
  a(1,1),a(2,2),a(3,3) : Selector  InputPortWidth=9  IndexOptions=Index vector (dialog)  Indices=[1 5 9]  OutputSizes=1
  a(1,1),a(2,3),a(3,2) : Selector  InputPortWidth=9  IndexOptions=Index vector (dialog)  Indices=[1 6 8]  OutputSizes=1
  a(1,2),a(2,1) : Selector  InputPortWidth=9  IndexOptions=Index vector (dialog)  Indices=[1 3]  OutputSizes=1
  a(1,2),a(2,1),a(3,3) : Selector  InputPortWidth=9  IndexOptions=Index vector (dialog)  Indices=[2 4 9]  OutputSizes=1
  a(1,2),a(2,3),a(3,1) : Selector  InputPortWidth=9  IndexOptions=Index vector (dialog)  Indices=[3 4 8]  OutputSizes=1
  a(1,3),a(2,1),a(3,2) : Selector  InputPortWidth=9  IndexOptions=Index vector (dialog)  Indices=[2 6 7]  OutputSizes=1
  a(1,3),a(2,2),a(3,1) : Selector  InputPortWidth=9  IndexOptions=Index vector (dialog)  Indices=[3 5 7]  OutputSizes=1
  a(1,3),a(3,1) : Selector  InputPortWidth=9  IndexOptions=Index vector (dialog)  Indices=[1 3]  OutputSizes=1
  a(1.1),a(3,3) : Selector  InputPortWidth=9  IndexOptions=Index vector (dialog)  Indices=[1 3]  OutputSizes=1
  a(2,2),a(3,3) : Selector  InputPortWidth=9  IndexOptions=Index vector (dialog)  Indices=[5 9]  OutputSizes=1
  a(3.2),a(2,3) : Selector  InputPortWidth=9  IndexOptions=Index vector (dialog)  Indices=[6 8]  OutputSizes=1
  I_SC : Outport
  R_Diag : Outport  Port=2
  wires:
  [I_SC_full] -> a(1,3),a(2,2),a(3,1)/1, a(1,3),a(2,1),a(3,2)/1, a(1,2),a(2,3),a(3,1)/1, a(1,1),a(2,2),a(3,3)/1, a(1,1),a(2,3),a(3,2)/1, a(1,2),a(2,1),a(3,3)/1
  Product2/1 -> Sum/3
  Product3/1 -> Sum/4
  a(1,2),a(2,1),a(3,3)/1 -> Product2/1
  a(1,1),a(2,3),a(3,2)/1 -> Product1/1
  Product/1 -> Sum/1
  a(1,3),a(2,2),a(3,1)/1 -> Product5/1
  a(1,1),a(2,2),a(3,3)/1 -> Product/1
  a(1,3),a(2,1),a(3,2)/1 -> Product4/1
  Product4/1 -> Sum/5
  Product1/1 -> Sum/2
  Product5/1 -> Sum/6
  a(1,2),a(2,3),a(3,1)/1 -> Product3/1
  I_SC_full/1 -> Reshape/1
  Reshape/1 -> [I_SC_full]
  Sum/1 -> [J3]  "det(I)"
  Product6/1 -> Sum1/1
  Product7/1 -> Sum1/2
  Product8/1 -> Sum1/3
  Sum1/1 -> [J2]  "I2"
  [I_SC_full] -> a(1,3),a(3,1)/1, a(1,1),a(2,2)/1, a(1,2),a(2,1)/1, a(1.1),a(3,3)/1, a(3.2),a(2,3)/1, a(2,2),a(3,3)/1
  [I_SC_full] -> Selector/1
  Selector/1 -> Sum of Elements/1
  a(2,2),a(3,3)/1 -> Product of Elements/1
  a(3.2),a(2,3)/1 -> Product of Elements1/1
  a(1.1),a(3,3)/1 -> Product of Elements2/1
  a(1,3),a(3,1)/1 -> Product of Elements3/1
  a(1,1),a(2,2)/1 -> Product of Elements4/1
  a(1,2),a(2,1)/1 -> Product of Elements5/1
  Product of Elements5/1 -> Product8/2
  Product of Elements4/1 -> Product8/1
  Product of Elements3/1 -> Product7/2
  Product of Elements2/1 -> Product7/1
  Product of Elements1/1 -> Product6/2
  Product of Elements/1 -> Product6/1
  Sum of Elements/1 -> [J1]  "tr(I)"
  [J2] -> Sum2/2
  [J1] -> Square/1
  Square/1 -> Gain2/1
  Gain2/1 -> Sum2/1
  Sum2/1 -> [p]
  [J2] -> Product10/2
  [J1] -> Product10/1
  [J3] -> Sum3/1
  Constant3/1 -> Power/2
  [J1] -> Power/1
  Power/1 -> Gain/1
  Product10/1 -> Gain1/1
  Gain1/1 -> Sum3/2
  Gain/1 -> Sum3/3
  Sum3/1 -> [q]
  [q] -> Square1/1
  [p] -> Power1/1
  Constant/1 -> Power1/2
  Square1/1 -> Gain4/1
  Power1/1 -> Gain3/1
  Gain4/1 -> Sum4/2
  Gain3/1 -> Sum4/1
  Sum4/1 -> Sqrt/1
  [q] -> Gain5/1
  Gain5/1 -> Sum5/2
  Sum5/1 -> Power2/1
  Constant1/1 -> Power2/2
  Power2/1 -> [u]
  Sqrt/1 -> [delta_3]
  [delta_3] -> Sum5/1
  [delta_3] -> Sum6/1
  Constant2/1 -> Power3/2
  Sum6/1 -> Power3/1
  [q] -> Gain6/1
  Power3/1 -> [v]
  Gain6/1 -> Sum6/2

== system Quaternions_Method_main/Inertia matrix/Main body ==
  m_MB : Inport
  a_MB : Inport  Port=2
  b_MB : Inport  Port=3
  h_MB : Inport  Port=4
  Constant : Constant  Value=0
  Gain : Gain  Gain=1/12
  Gain1 : Gain  Gain=1/12
  Gain2 : Gain  Gain=1/12
  Product : Product
  Product1 : Product
  Product2 : Product
  Reshape : Reshape  OutputDimensionality=Customize  OutputDimensions=[3,3]
  Square : Math  Operator=square  SaturateOnIntegerOverflow=on
  Square1 : Math  Operator=square  SaturateOnIntegerOverflow=on
  Square2 : Math  Operator=square  SaturateOnIntegerOverflow=on
  Sum : Sum
  Sum1 : Sum
  Sum2 : Sum
  Vector Concatenate : Concatenate  NumInputs=9
  I_MB : Outport
  wires:
  Constant/1 -> Vector Concatenate/2, Vector Concatenate/3, Vector Concatenate/7, Vector Concatenate/8, Vector Concatenate/6, Vector Concatenate/4
  Square/1 -> Sum2/1, Sum1/1
  Square1/1 -> Sum2/2, Sum/1
  Square2/1 -> Sum/2, Sum1/2
  Product1/1 -> Gain1/1
  Gain/1 -> Vector Concatenate/1
  Product2/1 -> Gain2/1
  Sum1/1 -> Product1/2
  m_MB/1 -> Product/1, Product2/1, Product1/1
  Sum2/1 -> Product2/2
  a_MB/1 -> Square/1
  Vector Concatenate/1 -> Reshape/1
  Sum/1 -> Product/2
  b_MB/1 -> Square1/1
  Gain1/1 -> Vector Concatenate/5
  Product/1 -> Gain/1
  Gain2/1 -> Vector Concatenate/9
  Reshape/1 -> I_MB/1
  h_MB/1 -> Square2/1

== system Quaternions_Method_main/Inertia matrix/SP_Rotation from SP principal to MB principal ==
  gamma_SP : Inport
  I_SP : Inport  Port=2
  Constant : Constant
  Demux : Demux  Outputs=9
  Gain : Gain  Gain=-1
  Gain1 : Gain  Gain=2
  Gain2 : Gain  Gain=1/2
  Ground : Ground
  Product : Product
  Reciprocal : Product  Inputs=/
  Reshape : Reshape  OutputDimensionality=Customize  OutputDimensions=[3,3]
  Sin : Trigonometry  Operator=cos
  Sin1 : Trigonometry
  Sin2 : Trigonometry  Operator=atan
  Sum : Sum  Inputs=+-
  Sum1 : Sum
  Terminator{,1..5} (6 alike) : Terminator
  Vector Concatenate : Concatenate  NumInputs=9
  R_SP : Outport
  alpha_P : Outport  Port=2
  wires:
  Vector Concatenate/1 -> Reshape/1
  Reshape/1 -> R_SP/1
  Constant/1 -> Vector Concatenate/1
  Ground/1 -> Vector Concatenate/7, Vector Concatenate/4, Vector Concatenate/3, Vector Concatenate/2
  gamma_SP/1 -> Sum1/1
  Gain/1 -> Vector Concatenate/6
  Sin/1 -> Vector Concatenate/5, Vector Concatenate/9
  Sin1/1 -> Gain/1, Vector Concatenate/8
  I_SP/1 -> Demux/1
  Demux/1 -> Terminator/1
  Demux/2 -> Terminator1/1
  Demux/3 -> Terminator2/1
  Demux/4 -> Terminator3/1
  Demux/5 -> Sum/1  "I22"
  Demux/6 -> Gain1/1  "I31"
  Demux/7 -> Terminator4/1
  Demux/8 -> Terminator5/1
  Demux/9 -> Sum/2  "I33"
  Sum/1 -> Reciprocal/1
  Reciprocal/1 -> Product/1
  Gain1/1 -> Product/2
  Product/1 -> Sin2/1
  Sin2/1 -> Gain2/1
  Gain2/1 -> alpha_P/1, Sum1/2
  Sum1/1 -> Sin1/1, Sin/1

== system Quaternions_Method_main/Inertia matrix/Solar panel ==
  note: The inertia matrix for the solar panels is for two solar panels since they are the same and they are on opposite sides the distance vector between the centers of mass are one the opposite of the other and in the transport theorem the sign does not matter since I need only the norm and the d'*d that has + sign anyway
      | Still the mass and all characteristics are about one solar panel
  m_SP : Inport
  a_SP : Inport  Port=2
  b_SP : Inport  Port=3
  h_SP : Inport  Port=4
  Gain : Gain  Gain=1/12
  Gain1 : Gain  Gain=1/12
  Gain2 : Gain  Gain=1/12
  Gain3 : Gain  Gain=2
  Ground : Ground
  Product : Product
  Product1 : Product
  Product2 : Product
  Reshape : Reshape  OutputDimensionality=Customize  OutputDimensions=[3,3]
  Square : Math  Operator=square  SaturateOnIntegerOverflow=on
  Square1 : Math  Operator=square  SaturateOnIntegerOverflow=on
  Square2 : Math  Operator=square  SaturateOnIntegerOverflow=on
  Sum : Sum
  Sum1 : Sum
  Sum2 : Sum
  Vector Concatenate : Concatenate  NumInputs=9
  I_SP : Outport
  wires:
  Vector Concatenate/1 -> Reshape/1
  m_SP/1 -> Product/1, Product2/1, Product1/1
  Product/1 -> Gain/1
  Gain/1 -> Vector Concatenate/1
  Product1/1 -> Gain1/1
  Product2/1 -> Gain2/1
  Gain2/1 -> Vector Concatenate/9
  h_SP/1 -> Square/1
  a_SP/1 -> Square1/1
  b_SP/1 -> Square2/1
  Sum/1 -> Product/2
  Sum1/1 -> Product1/2
  Sum2/1 -> Product2/2
  Ground/1 -> Vector Concatenate/2, Vector Concatenate/3, Vector Concatenate/7, Vector Concatenate/8, Vector Concatenate/6, Vector Concatenate/4
  Gain1/1 -> Vector Concatenate/5
  Reshape/1 -> Gain3/1
  Gain3/1 -> I_SP/1
  Square1/1 -> Sum1/2, Sum2/1
  Square2/1 -> Sum/2, Sum2/2
  Square/1 -> Sum/1, Sum1/1

== system Quaternions_Method_main/Inertia matrix/Transport theorem ==
  I_SP : Inport
  r_SP : Inport  Port=2
  m_SP : Inport  Port=3
  Constant : Constant  Value=eye(3)
  Dot Product : DotProduct  InputSameDT=on  OutDataTypeStr=Inherit: Inherit via internal rule
  Gain : Gain  Gain=2
  Matrix Multiply : Product  Multiplication=Matrix(*)
  Matrix Multiply1 : Product
  Product : Product
  Sum : Sum  Inputs=+-
  Sum1 : Sum
  Transpose : Math  Operator=transpose  SaturateOnIntegerOverflow=on
  I_SP_B : Outport
  wires:
  r_SP/1 -> Transpose/1, Dot Product/2, Dot Product/1, Matrix Multiply/2
  Transpose/1 -> Matrix Multiply/1
  Constant/1 -> Matrix Multiply1/1
  Matrix Multiply1/1 -> Sum/1
  Matrix Multiply/1 -> Sum/2
  Sum/1 -> Product/2
  m_SP/1 -> Gain/1
  Product/1 -> Sum1/2
  I_SP/1 -> Sum1/1
  Sum1/1 -> I_SP_B/1
  Dot Product/1 -> Matrix Multiply1/2
  Gain/1 -> Product/1

== system Quaternions_Method_main/Inertia matrix/gamma_SP ==
  R_diag : Inport
  S_B : Inport  Port=2
  Cos : Trigonometry  Operator=acos
  Demux : Demux  Outputs=3
  Gain : Gain  Gain=-1
  Matrix Multiply1 : Product  Multiplication=Matrix(*)
  Terminator : Terminator
  Terminator1 : Terminator
  gamma_SP : Outport
  wires:
  R_diag/1 -> Matrix Multiply1/1
  S_B/1 -> Matrix Multiply1/2
  Matrix Multiply1/1 -> Demux/1  "S_p_SP"
  Demux/1 -> Terminator/1
  Demux/2 -> Terminator1/1
  Demux/3 -> Gain/1
  Gain/1 -> Cos/1
  Cos/1 -> gamma_SP/1

== system Quaternions_Method_main/Inertia matrix/r_SP ==
  b_SP : Inport
  a_MB : Inport  Port=2
  Constant : Constant  Value=[1 0 0]
  Gain : Gain  Gain=1/2
  Gain1 : Gain  Gain=1/2
  Gain2 : Gain  Gain=-1
  Product : Product
  Reshape : Reshape  OutputDimensionality=Column vector (2-D)
  Sum : Sum
  r_SP1 : Outport
  r_SP2 : Outport  Port=2
  wires:
  Constant/1 -> Reshape/1
  a_MB/1 -> Gain/1
  b_SP/1 -> Gain1/1
  Gain1/1 -> Sum/1
  Gain/1 -> Sum/2
  Reshape/1 -> Product/1
  Sum/1 -> Product/2
  Gain2/1 -> r_SP2/1
  Product/1 -> r_SP1/1, Gain2/1

== system Quaternions_Method_main/Kalman Obs/Subsystem ==
  I_SC : Inport
  Demux1 : Demux  Outputs=9
  Divide3 : Product  Inputs=*/
  Divide4 : Product  Inputs=*/
  Divide5 : Product  Inputs=*/
  Mux1 : Mux  Inputs=3
  Reshape : Reshape  OutputDimensionality=Column vector (2-D)
  Sum3 : Sum  Inputs=|+-
  Sum4 : Sum  Inputs=|+-
  Sum5 : Sum  Inputs=|+-
  Terminator{,1..5} (6 alike) : Terminator
  K : Outport
  wires:
  Demux1/8 -> Terminator5/1
  Demux1/5 -> Divide3/2, Sum3/2, Sum4/1
  Demux1/3 -> Terminator1/1
  Reshape/1 -> Demux1/1
  Demux1/2 -> Terminator/1
  Demux1/1 -> Sum5/2, Divide5/2, Sum3/1
  Demux1/9 -> Divide4/2, Sum4/2, Sum5/1
  Demux1/4 -> Terminator2/1
  Demux1/7 -> Terminator4/1
  I_SC/1 -> Reshape/1
  Sum4/1 -> Divide5/1
  Sum3/1 -> Divide4/1
  Divide4/1 -> Mux1/3
  Divide5/1 -> Mux1/1
  Mux1/1 -> K/1
  Divide3/1 -> Mux1/2
  Demux1/6 -> Terminator3/1
  Sum5/1 -> Divide3/1

== system Quaternions_Method_main/Kalman Obs/Subsystem1 ==
  w_obs : Inport
  K : Inport  Port=2
  Demux : Demux  Outputs=3
  Demux1 : Demux  Outputs=3
  Ground : Ground
  Ground1 : Ground
  Ground2 : Ground
  Mux : Mux  Inputs=9
  Product{,1..5} (6 alike) : Product
  Reshape : Reshape  OutputDimensionality=Customize  OutputDimensions=[3,3]
  A : Outport
  wires:
  Reshape/1 -> A/1
  Mux/1 -> Reshape/1
  Demux/3 -> Product2/2, Product/2
  Product3/1 -> Mux/6
  Product4/1 -> Mux/7
  w_obs/1 -> Demux/1
  Demux1/1 -> Product1/1, Product/1
  Product5/1 -> Mux/8
  Ground2/1 -> Mux/9
  Demux1/3 -> Product5/1, Product4/1
  Product1/1 -> Mux/3
  Ground/1 -> Mux/1
  Product/1 -> Mux/2
  Product2/1 -> Mux/4
  K/1 -> Demux1/1
  Demux/2 -> Product4/2, Product1/2
  Demux1/2 -> Product2/1, Product3/1
  Ground1/1 -> Mux/5
  Demux/1 -> Product5/2, Product3/2

== system Quaternions_Method_main/Kalman Obs/Subsystem2 ==
  C : Inport
  P : Inport  Port=2
  R : Inport  Port=3
  Matrix Multiply : Product  Multiplication=Matrix(*)
  Matrix Multiply1 : Product  Multiplication=Matrix(*)
  Reciprocal : Product  Inputs=/  Multiplication=Matrix(*)
  Transpose : Math  Operator=transpose  SaturateOnIntegerOverflow=on
  L : Outport
  wires:
  Matrix Multiply1/1 -> L/1
  P/1 -> Matrix Multiply/1
  Transpose/1 -> Matrix Multiply/2
  C/1 -> Transpose/1
  Matrix Multiply/1 -> Matrix Multiply1/1
  R/1 -> Reciprocal/1
  Reciprocal/1 -> Matrix Multiply1/2

== system Quaternions_Method_main/Kalman Obs/Subsystem3 ==
  L : Inport
  w_m : Inport  Port=2
  C : Inport  Port=3
  w_obs : Inport  Port=4
  Demux : Demux  Outputs=9
  Demux1 : Demux  Outputs=3
  Demux2 : Demux  Outputs=3
  Matrix Multiply : Product  Multiplication=Matrix(*)
  Mux : Mux  Inputs=3
  Product : Product
  Product1 : Product
  Product2 : Product
  Reshape : Reshape  OutputDimensionality=Column vector (2-D)
  Sum : Sum  Inputs=|+-
  Sum1 : Sum  Inputs=|+-
  Sum2 : Sum  Inputs=|+-
  Terminator{,1..2,4..6} (6 alike) : Terminator
  Ly : Outport
  wires:
  w_obs/1 -> Demux2/1
  Matrix Multiply/1 -> Ly/1
  w_m/1 -> Demux1/1
  Demux/3 -> Terminator1/1
  Product2/1 -> Mux/3
  Product1/1 -> Mux/2
  Demux/1 -> Sum2/2
  Demux1/1 -> Sum2/1
  Demux/4 -> Terminator2/1
  Demux/2 -> Terminator/1
  Demux1/2 -> Sum/1
  Demux2/2 -> Product1/2
  Demux1/3 -> Sum1/1
  L/1 -> Matrix Multiply/1
  Mux/1 -> Matrix Multiply/2
  Demux2/1 -> Product/2
  Demux/8 -> Terminator6/1
  Sum1/1 -> Product2/1
  Demux/5 -> Sum/2
  Sum/1 -> Product1/1
  Demux/7 -> Terminator5/1
  Demux2/3 -> Product2/2
  Product/1 -> Mux/1
  Demux/9 -> Sum1/2
  Demux/6 -> Terminator4/1
  Reshape/1 -> Demux/1
  Sum2/1 -> Product/1
  C/1 -> Reshape/1

== system Quaternions_Method_main/Kalman Obs/Subsystem4 ==
  K : Inport
  w_obs : Inport  Port=2
  I_sc : Inport  Port=3
  hr_dot : Inport  Port=4
  Ly : Inport  Port=5
  Demux : Demux  Outputs=3
  Demux1 : Demux  Outputs=9
  Demux2 : Demux  Outputs=3
  Demux3 : Demux  Outputs=3
  Divide : Product  Inputs=*/
  Divide1 : Product  Inputs=*/
  Divide2 : Product  Inputs=*/
  Mux : Mux  Inputs=3
  Mux1 : Mux  Inputs=3
  Product{1..6} (6 alike) : Product
  Reshape : Reshape  OutputDimensionality=Column vector (2-D)
  Sum : Sum  Inputs=|++
  Sum1 : Sum  Inputs=|++
  Terminator{,1..5} (6 alike) : Terminator
  w_obs_dot : Outport
  wires:
  K/1 -> Demux/1
  w_obs/1 -> Demux3/1
  Ly/1 -> Sum1/2
  Demux/1 -> Product1/1
  Demux3/2 -> Product3/2, Product1/2
  Demux/2 -> Product2/1
  Demux/3 -> Product3/1
  Demux3/1 -> Product6/2, Product2/2
  Product1/1 -> Product4/1
  Product2/1 -> Product5/1
  Product3/1 -> Product6/1
  Demux3/3 -> Product5/2, Product4/2
  Product5/1 -> Mux/2
  Product4/1 -> Mux/1
  Product6/1 -> Mux/3
  Mux/1 -> Sum/1
  Sum/1 -> Sum1/1
  Sum1/1 -> w_obs_dot/1
  Demux1/4 -> Terminator2/1
  Divide1/1 -> Mux1/2
  Demux1/1 -> Divide/2
  Demux2/2 -> Divide1/1
  Demux1/6 -> Terminator3/1
  Divide/1 -> Mux1/1
  Mux1/1 -> Sum/2
  I_sc/1 -> Reshape/1
  Reshape/1 -> Demux1/1
  Demux1/7 -> Terminator4/1
  Demux1/9 -> Divide2/2
  Demux1/2 -> Terminator/1
  Demux2/3 -> Divide2/1
  Demux1/3 -> Terminator1/1
  Demux1/5 -> Divide1/2
  Divide2/1 -> Mux1/3
  Demux2/1 -> Divide/1
  Demux1/8 -> Terminator5/1
  hr_dot/1 -> Demux2/1

== system Quaternions_Method_main/Kalman Obs/Subsystem5 ==
  P : Inport
  A : Inport  Port=2
  Q : Inport  Port=3
  C : Inport  Port=4
  R : Inport  Port=5
  Matrix Multiply{,1..5} (6 alike) : Product  Multiplication=Matrix(*)
  Reciprocal : Product  Inputs=/  Multiplication=Matrix(*)
  Sum : Sum  Inputs=|++
  Sum1 : Sum  Inputs=|++
  Sum2 : Sum  Inputs=|+-
  Transpose : Math  Operator=transpose  SaturateOnIntegerOverflow=on
  Transpose1 : Math  Operator=transpose  SaturateOnIntegerOverflow=on
  P_dot : Outport
  wires:
  C/1 -> Transpose1/1
  Matrix Multiply2/1 -> Matrix Multiply3/1
  Sum1/1 -> Sum2/1
  Transpose/1 -> Matrix Multiply/2
  Transpose1/1 -> Matrix Multiply4/2, Matrix Multiply2/2
  R/1 -> Reciprocal/1
  Matrix Multiply3/1 -> Matrix Multiply4/1
  Matrix Multiply1/1 -> Sum/2
  Matrix Multiply4/1 -> Matrix Multiply5/1
  Matrix Multiply/1 -> Sum/1
  Matrix Multiply5/1 -> Sum2/2
  Sum/1 -> Sum1/1
  A/1 -> Matrix Multiply1/1, Transpose/1
  P/1 -> Matrix Multiply/1, Matrix Multiply2/1, Matrix Multiply5/2, Matrix Multiply1/2
  Sum2/1 -> P_dot/1
  Reciprocal/1 -> Matrix Multiply3/2
  [Q] -> Sum1/2
  Q/1 -> [Q]

== system Quaternions_Method_main/Kinematics1/Creazione Matrice A_BN ==
  q_normalizzato : Inport
  Reshape : Reshape  OutputDimensionality=Customize  OutputDimensions=[3,3]
  Vector Concatenate : Concatenate  NumInputs=3
  column 1 : Subsystem
  column 2 : Subsystem
  column 3 : Subsystem
  A_BN : Outport
  wires:
  Reshape/1 -> A_BN/1
  q_normalizzato/1 -> column 3/1(q_normalizzato), column 1/1(q_normalizzato), column 2/1(q_normalizzato)
  column 1/1(Column 1) -> Vector Concatenate/1
  column 2/1(Column 2) -> Vector Concatenate/2
  column 3/1(Column 3) -> Vector Concatenate/3
  Vector Concatenate/1 -> Reshape/1
